simulink model "QAM16WithNoise"  (R2014a)
settings: Solver=ode45  StartTime=0.0  StopTime=1.0  RelTol=1e-3
libraries: commchan3 x1, commrflib2 x1, commrandsrc2 x1, commdigbbndam3 x1
settings Model: Creator=okuu  LastModifiedBy=okuu

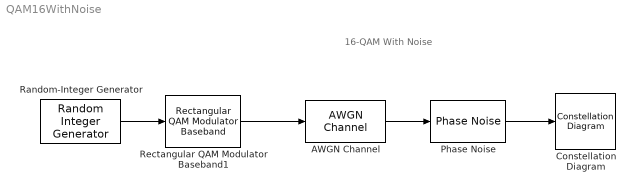
== system QAM16WithNoise ==
  note: 16-QAM With Noise
  AWGN Channel : commchan3/AWGN Channel  InputProcessing=Columns as channels (frame based)  seed=1337  noiseMode="Signal to noise ratio  (Es/No)"  EbNodB=10  EsNodB=30  SNRdB=10  bitsPerSym=1  Ps=1  Tsym=.01  variance=1
  Constellation Diagram : ConstellationDiagram
  Phase Noise : commrflib2/Phase Noise  PhNs=-70  Fo=200  Fs=1024  seed=7331
  Random-Integer Generator : commrandsrc2/Random Integer Generator  mul=16  seed=1337  Ts=.01  frameBased=on  sampPerFrame=1000  orient=off  outDataType=uint8
  Rectangular QAM Modulator Baseband1 : commdigbbndam3/Rectangular QAM Modulator Baseband  M=16  InType=Integer  Enc=Gray  Mapping=[0:15]  PowType=Average Power  MinDist=2  AvgPow=1  PeakPow=1  Ph=0  outDtype=single  outWordLen=16  outUDDataType=sfix(16)  outFracLenMode=Best precision  outFracLen=15
  wires:
  Phase Noise/1 -> Constellation Diagram/1
  Random-Integer Generator/1 -> Rectangular QAM Modulator Baseband1/1
  Rectangular QAM Modulator Baseband1/1 -> AWGN Channel/1
  AWGN Channel/1 -> Phase Noise/1
